simulink model "sub32_4n_model_run"  (R2023b)
settings: Solver=VariableStepAuto  StartTime=0.0  StopTime=5000E-12  FixedStep=1e-20  RelTol=1e-3
model workspace (MAT data in the model file):
  tp_delay = 1.25e-10
values from neighbouring files (symbols this model uses):
  tp_combinerA1_G8 = mean_CtoG + normrnd(0, stdev_CtoG)    [blockConf.m]
  tp_combinerA2_G4 = mean_CtoG + normrnd(0, stdev_CtoG)    [blockConf.m]
  tp_combinerA3_G2 = mean_CtoG + normrnd(0, stdev_CtoG)    [blockConf.m]
  tp_combinerA4_G1 = mean_CtoG + normrnd(0, stdev_CtoG)    [blockConf.m]
  tp_combinerB1_G8 = mean_CtoG + normrnd(0, stdev_CtoG)    [blockConf.m]
  tp_combinerB2_G4 = mean_CtoG + normrnd(0, stdev_CtoG)    [blockConf.m]
  tp_combinerB3_G2 = mean_CtoG + normrnd(0, stdev_CtoG)    [blockConf.m]
  tp_combinerB4_G1 = mean_CtoG + normrnd(0, stdev_CtoG)    [blockConf.m]
  tp_delay_1 = mean_DtoR + normrnd(0, stdev_DtoR)    [blockConf.m]
  tp_delay_10 = mean_DtoR + normrnd(0, stdev_DtoR)    [blockConf.m]
  tp_delay_11 = mean_DtoR + normrnd(0, stdev_DtoR)    [blockConf.m]
  tp_delay_12 = mean_DtoR + normrnd(0, stdev_DtoR)    [blockConf.m]
  tp_delay_13 = mean_DtoR + normrnd(0, stdev_DtoR)    [blockConf.m]
  tp_delay_14 = mean_DtoR + normrnd(0, stdev_DtoR)    [blockConf.m]
  tp_delay_15 = mean_DtoR + normrnd(0, stdev_DtoR)    [blockConf.m]
  tp_delay_16 = mean_DtoR + normrnd(0, stdev_DtoR)    [blockConf.m]
  tp_delay_17 = mean_DtoR + normrnd(0, stdev_DtoR)    [blockConf.m]
  tp_delay_18 = mean_DtoR + normrnd(0, stdev_DtoR)    [blockConf.m]
  tp_delay_19 = mean_DtoR + normrnd(0, stdev_DtoR)    [blockConf.m]
  tp_delay_2 = mean_DtoR + normrnd(0, stdev_DtoR)    [blockConf.m]
  tp_delay_20 = mean_DtoR + normrnd(0, stdev_DtoR)    [blockConf.m]
  tp_delay_21 = mean_DtoR + normrnd(0, stdev_DtoR)    [blockConf.m]
  tp_delay_22 = mean_DtoR + normrnd(0, stdev_DtoR)    [blockConf.m]
  tp_delay_23 = mean_DtoR + normrnd(0, stdev_DtoR)    [blockConf.m]
  tp_delay_24 = mean_DtoR + normrnd(0, stdev_DtoR)    [blockConf.m]
  tp_delay_25 = mean_DtoR + normrnd(0, stdev_DtoR)    [blockConf.m]
  tp_delay_26 = mean_DtoR + normrnd(0, stdev_DtoR)    [blockConf.m]
  tp_delay_27 = mean_DtoR + normrnd(0, stdev_DtoR)    [blockConf.m]
  tp_delay_28 = mean_DtoR + normrnd(0, stdev_DtoR)    [blockConf.m]
  tp_delay_29 = mean_DtoR + normrnd(0, stdev_DtoR)    [blockConf.m]
  tp_delay_3 = mean_DtoR + normrnd(0, stdev_DtoR)    [blockConf.m]
  tp_delay_30 = mean_DtoR + normrnd(0, stdev_DtoR)    [blockConf.m]
  tp_delay_31 = mean_DtoR + normrnd(0, stdev_DtoR)    [blockConf.m]
  tp_delay_32 = mean_DtoR + normrnd(0, stdev_DtoR)    [blockConf.m]
  tp_delay_4 = mean_DtoR + normrnd(0, stdev_DtoR)    [blockConf.m]
  tp_delay_5 = mean_DtoR + normrnd(0, stdev_DtoR)    [blockConf.m]
  tp_delay_6 = mean_DtoR + normrnd(0, stdev_DtoR)    [blockConf.m]
  tp_delay_7 = mean_DtoR + normrnd(0, stdev_DtoR)    [blockConf.m]
  tp_delay_8 = mean_DtoR + normrnd(0, stdev_DtoR)    [blockConf.m]
  tp_delay_9 = mean_DtoR + normrnd(0, stdev_DtoR)    [blockConf.m]
  tp_delay_b1 = mean_delay + normrnd(0, stdev_delay)    [blockConf.m]
  tp_delay_b10 = mean_delay + normrnd(0, stdev_delay)    [blockConf.m]
  tp_delay_b11 = mean_delay + normrnd(0, stdev_delay)    [blockConf.m]
  tp_delay_b12 = mean_delay + normrnd(0, stdev_delay)    [blockConf.m]
  tp_delay_b13 = mean_delay + normrnd(0, stdev_delay)    [blockConf.m]
  tp_delay_b14 = mean_delay + normrnd(0, stdev_delay)    [blockConf.m]
  tp_delay_b15 = mean_delay + normrnd(0, stdev_delay)    [blockConf.m]
  tp_delay_b16 = mean_delay + normrnd(0, stdev_delay)    [blockConf.m]
  tp_delay_b17 = mean_delay + normrnd(0, stdev_delay)    [blockConf.m]
  tp_delay_b18 = mean_delay + normrnd(0, stdev_delay)    [blockConf.m]
  tp_delay_b19 = mean_delay + normrnd(0, stdev_delay)    [blockConf.m]
  tp_delay_b2 = mean_delay + normrnd(0, stdev_delay)    [blockConf.m]
  tp_delay_b20 = mean_delay + normrnd(0, stdev_delay)    [blockConf.m]
  tp_delay_b21 = mean_delay + normrnd(0, stdev_delay)    [blockConf.m]
  tp_delay_b22 = mean_delay + normrnd(0, stdev_delay)    [blockConf.m]
  tp_delay_b23 = mean_delay + normrnd(0, stdev_delay)    [blockConf.m]
  tp_delay_b24 = mean_delay + normrnd(0, stdev_delay)    [blockConf.m]
  tp_delay_b25 = mean_delay + normrnd(0, stdev_delay)    [blockConf.m]
  tp_delay_b26 = mean_delay + normrnd(0, stdev_delay)    [blockConf.m]
  tp_delay_b27 = mean_delay + normrnd(0, stdev_delay)    [blockConf.m]
  tp_delay_b28 = mean_delay + normrnd(0, stdev_delay)    [blockConf.m]
  tp_delay_b29 = mean_delay + normrnd(0, stdev_delay)    [blockConf.m]
  tp_delay_b3 = mean_delay + normrnd(0, stdev_delay)    [blockConf.m]
  tp_delay_b30 = mean_delay + normrnd(0, stdev_delay)    [blockConf.m]
  tp_delay_b31 = mean_delay + normrnd(0, stdev_delay)    [blockConf.m]
  tp_delay_b4 = mean_delay + normrnd(0, stdev_delay)    [blockConf.m]
  tp_delay_b5 = mean_delay + normrnd(0, stdev_delay)    [blockConf.m]
  tp_delay_b6 = mean_delay + normrnd(0, stdev_delay)    [blockConf.m]
  tp_delay_b7 = mean_delay + normrnd(0, stdev_delay)    [blockConf.m]
  tp_delay_b8 = mean_delay + normrnd(0, stdev_delay)    [blockConf.m]
  tp_delay_b9 = mean_delay + normrnd(0, stdev_delay)    [blockConf.m]
  tp_pa_1 = mean_GtoP + normrnd(0, stdev_GtoP1)    [blockConf.m]
  tp_pa_2 = mean_GtoP + normrnd(0, stdev_GtoP2)    [blockConf.m]
  tp_pa_3 = mean_GtoP + normrnd(0, stdev_GtoP3)    [blockConf.m]
  tp_pa_4 = mean_GtoP + normrnd(0, stdev_GtoP4)    [blockConf.m]
  tp_router10_1 = mean_RtoC + normrnd(0, stdev_RtoC)    [blockConf.m]
  tp_router10_2 = mean_RtoC + normrnd(0, stdev_RtoC)    [blockConf.m]
  tp_router10_4 = mean_RtoC + normrnd(0, stdev_RtoC)    [blockConf.m]
  tp_router10_8 = mean_RtoC + normrnd(0, stdev_RtoC)    [blockConf.m]
  tp_router11_1 = mean_RtoC + normrnd(0, stdev_RtoC)    [blockConf.m]
  tp_router11_2 = mean_RtoC + normrnd(0, stdev_RtoC)    [blockConf.m]
  tp_router11_4 = mean_RtoC + normrnd(0, stdev_RtoC)    [blockConf.m]
  tp_router11_8 = mean_RtoC + normrnd(0, stdev_RtoC)    [blockConf.m]
  tp_router12_1 = mean_RtoC + normrnd(0, stdev_RtoC)    [blockConf.m]
  tp_router12_2 = mean_RtoC + normrnd(0, stdev_RtoC)    [blockConf.m]
  tp_router12_4 = mean_RtoC + normrnd(0, stdev_RtoC)    [blockConf.m]
  tp_router12_8 = mean_RtoC + normrnd(0, stdev_RtoC)    [blockConf.m]
  tp_router13_1 = mean_RtoC + normrnd(0, stdev_RtoC)    [blockConf.m]
  tp_router13_2 = mean_RtoC + normrnd(0, stdev_RtoC)    [blockConf.m]
  tp_router13_4 = mean_RtoC + normrnd(0, stdev_RtoC)    [blockConf.m]
  tp_router13_8 = mean_RtoC + normrnd(0, stdev_RtoC)    [blockConf.m]
  tp_router14_1 = mean_RtoC + normrnd(0, stdev_RtoC)    [blockConf.m]
  tp_router14_2 = mean_RtoC + normrnd(0, stdev_RtoC)    [blockConf.m]
  tp_router14_4 = mean_RtoC + normrnd(0, stdev_RtoC)    [blockConf.m]
  tp_router14_8 = mean_RtoC + normrnd(0, stdev_RtoC)    [blockConf.m]
  tp_router15_1 = mean_RtoC + normrnd(0, stdev_RtoC)    [blockConf.m]
  tp_router15_2 = mean_RtoC + normrnd(0, stdev_RtoC)    [blockConf.m]
  tp_router15_4 = mean_RtoC + normrnd(0, stdev_RtoC)    [blockConf.m]
  tp_router15_8 = mean_RtoC + normrnd(0, stdev_RtoC)    [blockConf.m]
  tp_router16_1 = mean_RtoC + normrnd(0, stdev_RtoC)    [blockConf.m]
  tp_router16_2 = mean_RtoC + normrnd(0, stdev_RtoC)    [blockConf.m]
  tp_router16_4 = mean_RtoC + normrnd(0, stdev_RtoC)    [blockConf.m]
  tp_router16_8 = mean_RtoC + normrnd(0, stdev_RtoC)    [blockConf.m]
  tp_router17_1 = mean_RtoC + normrnd(0, stdev_RtoC)    [blockConf.m]
  tp_router17_2 = mean_RtoC + normrnd(0, stdev_RtoC)    [blockConf.m]
  tp_router17_4 = mean_RtoC + normrnd(0, stdev_RtoC)    [blockConf.m]
  tp_router17_8 = mean_RtoC + normrnd(0, stdev_RtoC)    [blockConf.m]
  tp_router18_1 = mean_RtoC + normrnd(0, stdev_RtoC)    [blockConf.m]
  tp_router18_2 = mean_RtoC + normrnd(0, stdev_RtoC)    [blockConf.m]
  tp_router18_4 = mean_RtoC + normrnd(0, stdev_RtoC)    [blockConf.m]
  tp_router18_8 = mean_RtoC + normrnd(0, stdev_RtoC)    [blockConf.m]
  tp_router19_1 = mean_RtoC + normrnd(0, stdev_RtoC)    [blockConf.m]
  tp_router19_2 = mean_RtoC + normrnd(0, stdev_RtoC)    [blockConf.m]
  tp_router19_4 = mean_RtoC + normrnd(0, stdev_RtoC)    [blockConf.m]
  tp_router19_8 = mean_RtoC + normrnd(0, stdev_RtoC)    [blockConf.m]
  tp_router1_1 = mean_RtoC + normrnd(0, stdev_RtoC)    [blockConf.m]
  tp_router1_2 = mean_RtoC + normrnd(0, stdev_RtoC)    [blockConf.m]
  tp_router1_4 = mean_RtoC + normrnd(0, stdev_RtoC)    [blockConf.m]
  tp_router1_8 = mean_RtoC + normrnd(0, stdev_RtoC)    [blockConf.m]
  tp_router20_1 = mean_RtoC + normrnd(0, stdev_RtoC)    [blockConf.m]
  ... (+83 more)
undefined symbols (not defined in the file or in its folder): r10_1, r10_2, r10_4, r10_8, r11_1, r11_2, r11_4, r11_8, r12_1, r12_2, r12_4, r12_8, r13_1, r13_2, r13_4, r13_8, r14_1, r14_2, r14_4, r14_8, r15_1, r15_2, r15_4, r15_8, r16_1, r16_2, r16_4, r16_8, r1_1, r1_2, r1_4, r1_8, r2_1, r2_2, r2_4, r2_8, r3_1, r3_2, r3_4, r3_8, r4_1, r4_2, r4_4, r4_8, r5_1, r5_2, r5_4, r5_8, r6_1, r6_2, r6_4, r6_8, r7_1, r7_2, r7_4, r7_8, r8_1, r8_2, r8_4, r8_8 ... (+4)
libraries: fl_lib x15, nesl_utility x3, simulink x2
(part 2 of 2)

== system sub32_4n_model_run/Subsystem29 ==
  In1 : Inport
  Gain : Gain  Gain=r5_1
  Gain1 : Gain  Gain=r5_2
  Gain2 : Gain  Gain=r5_4
  Gain3 : Gain  Gain=r5_8
  Transport Delay : TransportDelay  DelayTime=tp_router28_1
  Transport Delay1 : TransportDelay  DelayTime=tp_router28_2
  Transport Delay2 : TransportDelay  DelayTime=tp_router28_4
  Transport Delay3 : TransportDelay  DelayTime=tp_router28_8
  Out1 : Outport
  Out2 : Outport  Port=2
  Out3 : Outport  Port=3
  Out4 : Outport  Port=4
  wires:
  Gain/1 -> Transport Delay/1
  Gain3/1 -> Transport Delay3/1
  Gain1/1 -> Transport Delay1/1
  In1/1 -> Gain1/1, Gain/1, Gain3/1, Gain2/1
  Gain2/1 -> Transport Delay2/1
  Transport Delay/1 -> Out1/1
  Transport Delay1/1 -> Out2/1
  Transport Delay2/1 -> Out3/1
  Transport Delay3/1 -> Out4/1

== system sub32_4n_model_run/Subsystem3 ==
  In1 : Inport
  Gain : Gain  Gain=r14_1
  Gain1 : Gain  Gain=r14_2
  Gain2 : Gain  Gain=r14_4
  Gain3 : Gain  Gain=r14_8
  Transport Delay : TransportDelay  DelayTime=tp_router14_1
  Transport Delay1 : TransportDelay  DelayTime=tp_router14_2
  Transport Delay2 : TransportDelay  DelayTime=tp_router14_4
  Transport Delay3 : TransportDelay  DelayTime=tp_router14_8
  Out1 : Outport
  Out2 : Outport  Port=2
  Out3 : Outport  Port=3
  Out4 : Outport  Port=4
  wires:
  Gain/1 -> Transport Delay/1
  Gain3/1 -> Transport Delay3/1
  Gain1/1 -> Transport Delay1/1
  In1/1 -> Gain1/1, Gain/1, Gain3/1, Gain2/1
  Gain2/1 -> Transport Delay2/1
  Transport Delay/1 -> Out1/1
  Transport Delay1/1 -> Out2/1
  Transport Delay2/1 -> Out3/1
  Transport Delay3/1 -> Out4/1

== system sub32_4n_model_run/Subsystem30 ==
  In1 : Inport
  Gain : Gain  Gain=r6_1
  Gain1 : Gain  Gain=r6_2
  Gain2 : Gain  Gain=r6_4
  Gain3 : Gain  Gain=r6_8
  Transport Delay : TransportDelay  DelayTime=tp_router27_1
  Transport Delay1 : TransportDelay  DelayTime=tp_router27_2
  Transport Delay2 : TransportDelay  DelayTime=tp_router27_4
  Transport Delay3 : TransportDelay  DelayTime=tp_router27_8
  Out1 : Outport
  Out2 : Outport  Port=2
  Out3 : Outport  Port=3
  Out4 : Outport  Port=4
  wires:
  Gain/1 -> Transport Delay/1
  Gain3/1 -> Transport Delay3/1
  Gain1/1 -> Transport Delay1/1
  In1/1 -> Gain1/1, Gain/1, Gain3/1, Gain2/1
  Gain2/1 -> Transport Delay2/1
  Transport Delay/1 -> Out1/1
  Transport Delay1/1 -> Out2/1
  Transport Delay2/1 -> Out3/1
  Transport Delay3/1 -> Out4/1

== system sub32_4n_model_run/Subsystem31 ==
  In1 : Inport
  Gain : Gain  Gain=r7_1
  Gain1 : Gain  Gain=r7_2
  Gain2 : Gain  Gain=r7_4
  Gain3 : Gain  Gain=r7_8
  Transport Delay : TransportDelay  DelayTime=tp_router26_1
  Transport Delay1 : TransportDelay  DelayTime=tp_router26_2
  Transport Delay2 : TransportDelay  DelayTime=tp_router26_4
  Transport Delay3 : TransportDelay  DelayTime=tp_router26_8
  Out1 : Outport
  Out2 : Outport  Port=2
  Out3 : Outport  Port=3
  Out4 : Outport  Port=4
  wires:
  Gain/1 -> Transport Delay/1
  Gain3/1 -> Transport Delay3/1
  Gain1/1 -> Transport Delay1/1
  In1/1 -> Gain1/1, Gain/1, Gain3/1, Gain2/1
  Gain2/1 -> Transport Delay2/1
  Transport Delay/1 -> Out1/1
  Transport Delay1/1 -> Out2/1
  Transport Delay2/1 -> Out3/1
  Transport Delay3/1 -> Out4/1

== system sub32_4n_model_run/Subsystem32 ==
  In1 : Inport
  Gain : Gain  Gain=r8_1
  Gain1 : Gain  Gain=r8_2
  Gain2 : Gain  Gain=r8_4
  Gain3 : Gain  Gain=r8_8
  Transport Delay : TransportDelay  DelayTime=tp_router25_1
  Transport Delay1 : TransportDelay  DelayTime=tp_router25_2
  Transport Delay2 : TransportDelay  DelayTime=tp_router25_4
  Transport Delay3 : TransportDelay  DelayTime=tp_router25_8
  Out1 : Outport
  Out2 : Outport  Port=2
  Out3 : Outport  Port=3
  Out4 : Outport  Port=4
  wires:
  Gain/1 -> Transport Delay/1
  Gain3/1 -> Transport Delay3/1
  Gain1/1 -> Transport Delay1/1
  In1/1 -> Gain1/1, Gain/1, Gain3/1, Gain2/1
  Gain2/1 -> Transport Delay2/1
  Transport Delay/1 -> Out1/1
  Transport Delay1/1 -> Out2/1
  Transport Delay2/1 -> Out3/1
  Transport Delay3/1 -> Out4/1

== system sub32_4n_model_run/Subsystem4 ==
  In1 : Inport
  Gain : Gain  Gain=r13_1
  Gain1 : Gain  Gain=r13_2
  Gain2 : Gain  Gain=r13_4
  Gain3 : Gain  Gain=r13_8
  Transport Delay : TransportDelay  DelayTime=tp_router13_1
  Transport Delay1 : TransportDelay  DelayTime=tp_router13_2
  Transport Delay2 : TransportDelay  DelayTime=tp_router13_4
  Transport Delay3 : TransportDelay  DelayTime=tp_router13_8
  Out1 : Outport
  Out2 : Outport  Port=2
  Out3 : Outport  Port=3
  Out4 : Outport  Port=4
  wires:
  Gain/1 -> Transport Delay/1
  Gain3/1 -> Transport Delay3/1
  Gain1/1 -> Transport Delay1/1
  In1/1 -> Gain1/1, Gain/1, Gain3/1, Gain2/1
  Gain2/1 -> Transport Delay2/1
  Transport Delay/1 -> Out1/1
  Transport Delay1/1 -> Out2/1
  Transport Delay2/1 -> Out3/1
  Transport Delay3/1 -> Out4/1

== system sub32_4n_model_run/Subsystem5 ==
  In1 : Inport
  Gain : Gain  Gain=r12_1
  Gain1 : Gain  Gain=r12_2
  Gain2 : Gain  Gain=r12_4
  Gain3 : Gain  Gain=r12_8
  Transport Delay : TransportDelay  DelayTime=tp_router12_1
  Transport Delay1 : TransportDelay  DelayTime=tp_router12_2
  Transport Delay2 : TransportDelay  DelayTime=tp_router12_4
  Transport Delay3 : TransportDelay  DelayTime=tp_router12_8
  Out1 : Outport
  Out2 : Outport  Port=2
  Out3 : Outport  Port=3
  Out4 : Outport  Port=4
  wires:
  Gain/1 -> Transport Delay/1
  Gain3/1 -> Transport Delay3/1
  Gain1/1 -> Transport Delay1/1
  In1/1 -> Gain1/1, Gain/1, Gain3/1, Gain2/1
  Gain2/1 -> Transport Delay2/1
  Transport Delay/1 -> Out1/1
  Transport Delay1/1 -> Out2/1
  Transport Delay2/1 -> Out3/1
  Transport Delay3/1 -> Out4/1

== system sub32_4n_model_run/Subsystem6 ==
  In1 : Inport
  Gain : Gain  Gain=r11_1
  Gain1 : Gain  Gain=r11_2
  Gain2 : Gain  Gain=r11_4
  Gain3 : Gain  Gain=r11_8
  Transport Delay : TransportDelay  DelayTime=tp_router11_1
  Transport Delay1 : TransportDelay  DelayTime=tp_router11_2
  Transport Delay2 : TransportDelay  DelayTime=tp_router11_4
  Transport Delay3 : TransportDelay  DelayTime=tp_router11_8
  Out1 : Outport
  Out2 : Outport  Port=2
  Out3 : Outport  Port=3
  Out4 : Outport  Port=4
  wires:
  Gain/1 -> Transport Delay/1
  Gain3/1 -> Transport Delay3/1
  Gain1/1 -> Transport Delay1/1
  In1/1 -> Gain1/1, Gain/1, Gain3/1, Gain2/1
  Gain2/1 -> Transport Delay2/1
  Transport Delay/1 -> Out1/1
  Transport Delay1/1 -> Out2/1
  Transport Delay2/1 -> Out3/1
  Transport Delay3/1 -> Out4/1

== system sub32_4n_model_run/Subsystem7 ==
  In1 : Inport
  Gain : Gain  Gain=r10_1
  Gain1 : Gain  Gain=r10_2
  Gain2 : Gain  Gain=r10_4
  Gain3 : Gain  Gain=r10_8
  Transport Delay : TransportDelay  DelayTime=tp_router10_1
  Transport Delay1 : TransportDelay  DelayTime=tp_router10_2
  Transport Delay2 : TransportDelay  DelayTime=tp_router10_4
  Transport Delay3 : TransportDelay  DelayTime=tp_router10_8
  Out1 : Outport
  Out2 : Outport  Port=2
  Out3 : Outport  Port=3
  Out4 : Outport  Port=4
  wires:
  Gain/1 -> Transport Delay/1
  Gain3/1 -> Transport Delay3/1
  Gain1/1 -> Transport Delay1/1
  In1/1 -> Gain1/1, Gain/1, Gain3/1, Gain2/1
  Gain2/1 -> Transport Delay2/1
  Transport Delay/1 -> Out1/1
  Transport Delay1/1 -> Out2/1
  Transport Delay2/1 -> Out3/1
  Transport Delay3/1 -> Out4/1

== system sub32_4n_model_run/Subsystem8 ==
  In1 : Inport
  Gain : Gain  Gain=r9_1
  Gain1 : Gain  Gain=r9_2
  Gain2 : Gain  Gain=r9_4
  Gain3 : Gain  Gain=r9_8
  Transport Delay : TransportDelay  DelayTime=tp_router9_1
  Transport Delay1 : TransportDelay  DelayTime=tp_router9_2
  Transport Delay2 : TransportDelay  DelayTime=tp_router9_4
  Transport Delay3 : TransportDelay  DelayTime=tp_router9_8
  Out1 : Outport
  Out2 : Outport  Port=2
  Out3 : Outport  Port=3
  Out4 : Outport  Port=4
  wires:
  Gain/1 -> Transport Delay/1
  Gain3/1 -> Transport Delay3/1
  Gain1/1 -> Transport Delay1/1
  In1/1 -> Gain1/1, Gain/1, Gain3/1, Gain2/1
  Gain2/1 -> Transport Delay2/1
  Transport Delay/1 -> Out1/1
  Transport Delay1/1 -> Out2/1
  Transport Delay2/1 -> Out3/1
  Transport Delay3/1 -> Out4/1

== system sub32_4n_model_run/Subsystem9 ==
  In1 : Inport
  Gain : Gain  Gain=r1_1
  Gain1 : Gain  Gain=r1_2
  Gain2 : Gain  Gain=r1_4
  Gain3 : Gain  Gain=r1_8
  Transport Delay : TransportDelay  DelayTime=tp_router32_1
  Transport Delay1 : TransportDelay  DelayTime=tp_router32_2
  Transport Delay2 : TransportDelay  DelayTime=tp_router32_4
  Transport Delay3 : TransportDelay  DelayTime=tp_router32_8
  Out1 : Outport
  Out2 : Outport  Port=2
  Out3 : Outport  Port=3
  Out4 : Outport  Port=4
  wires:
  Gain/1 -> Transport Delay/1
  Gain3/1 -> Transport Delay3/1
  Gain1/1 -> Transport Delay1/1
  In1/1 -> Gain1/1, Gain/1, Gain3/1, Gain2/1
  Gain2/1 -> Transport Delay2/1
  Transport Delay/1 -> Out1/1
  Transport Delay1/1 -> Out2/1
  Transport Delay2/1 -> Out3/1
  Transport Delay3/1 -> Out4/1
